simulink model "New_prop_post_tequila"  (R2020b)
settings: Solver=VariableStepAuto  StartTime=0.0  StopTime=10.0  RelTol=1e-3
settings Model: Creator=Jonathan van Zyl  LastModifiedBy=Jonathan van Zyl

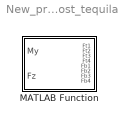
== system New_prop_post_tequila ==
  MATLAB Function : MATLAB Function  TreatAsAtomicUnit=on

== matlab function New_prop_post_tequila/MATLAB Function ==
  data: My input; Ft1 output; Fz input; Ft2 output; Ft3 output; Ft4 output; Fb1 output; Fb2 output; Fb3 output; Fb4 output
function [Ft1, Ft2, Ft3, Ft4, Fb1, Fb2, Fb3, Fb4] = fixingpropulsionsmess(My, Fz)
xt_1 = 1.2598;
xb_1 = 2.2598;
xt_3 = -1.3402;
x_t1 = xt_1;
x_b1 = xb_1;
x_t3 = xt_3;

alpha_1 = (-2*xt_1*(1/((xt_1/xb_1)-1))*(2 - (2*xb_3/xb_1)) - 4*xb_3)^2;
alpha_2 = ((1/((xt_1/xb_1)-1))*(2-(2*xb_3/xb_1)))^2;
alpha = alpha_1 + alpha_2;

beta_1 = 2*My*((1/(2*xb_1))*(1 - (xt_1/xb_1)*(1/((xt_1/xb_1) -1))));
beta_2 = 2*My*(1/((xt_1/xb_1) -1))*(1/(2*xb_1))*(1/((xt_1/xb_1) -1))*(2 - ((2*xb_3)/x_b1));



y = u;
